simulink model "pcssp_TF"  (R2020b)
settings: configuration reference "configurationSettings" (kept outside this file)
values from neighbouring files (symbols this model uses):
  pcssp_TF_fp = 0.0    [pcssp_TF.sldd]
undefined symbols (not defined in the file or in its folder): pcssp_TF_tp
settings Model: DataDictionary=pcssp_TF.sldd  Creator=ravenst1  LastModifiedBy=timoravensbergen
settings ConfigSetRef: SourceName=configurationSettings

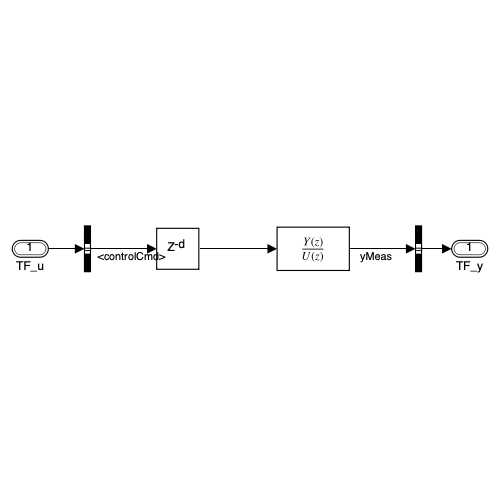
[thumbnail: Simulink's stored preview of the top-level diagram]
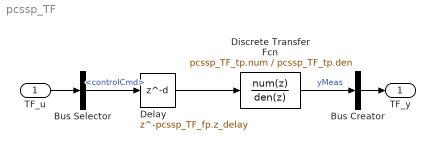
== system pcssp_TF ==
  TF_u : Inport  OutDataTypeStr=Bus: pcssp_TF_inBus  SampleTime=pcssp_TF_fp.timing.dt
  Bus Creator : BusCreator  Inputs=1  OutDataTypeStr=Bus: pcssp_TF_outBus
  Bus Selector : BusSelector  OutputSignals=controlCmd
  Delay : Delay  DelayLength=pcssp_TF_fp.z_delay
  Discrete Transfer Fcn : DiscreteTransferFcn  Numerator=pcssp_TF_tp.num  Denominator=pcssp_TF_tp.den
  TF_y : Outport  OutDataTypeStr=Bus: pcssp_TF_outBus
  wires:
  Delay/1 -> Discrete Transfer Fcn/1
  Discrete Transfer Fcn/1 -> Bus Creator/1  "yMeas"
  TF_u/1 -> Bus Selector/1
  Bus Selector/1 -> Delay/1  "<controlCmd>"
  Bus Creator/1 -> TF_y/1
